simulink model "MMSAR_Sequential2019"  (R2019b)
settings: Solver=VariableStepAuto  StartTime=0.0  StopTime=2.85  RelTol=1e-3
values from neighbouring files (symbols this model uses):
  ADC_input = database_load('EEGdata_ch1.mat',p)'    [MMSeq_main.m]    (also in database_load.m = data(:, epoch))
  C2 = C1*cap_ratio    [MMSeq_main.m]
  Cf_unit_cap = 2    [MMSeq_main.m]
  clk_freq = 2.1*input_BW    (= 537.6)    [MMSeq_main.m]
  clk_period = 1/clk_freq    (= 0.00186011904762)    [MMSeq_main.m]
  comparator_high_offset = 655e-6    (= 0.000655)    [MMSeq_main.m]
  comparator_low_offset = comparator_high_offset    (= 0.000655)    [MMSeq_main.m]
  comparator_noise_on = 1    [MMSeq_main.m]
  comparator_noise_rms = noise_multiplier* 1*sqrt(k*T/C_logic * (2/3))    [MMSeq_main.m]
  comparator_offset_on = 1    [MMSeq_main.m]
  DAC_cap = max([minimum_sampling_cap, minimum_technology_cap, minimum_match_cap_DAC])    [MMSeq_main.m]
  k = 1.38064852e-23    [MMSeq_main.m]
  leak_current = leakage_on *1*10^(-15)    (= 1e-15)    [MMSeq_main.m]
  LNA_bandwidth = 3*input_BW    (= 768)    [MMSeq_main.m]
  LNA_gain = 1000    [MMSeq_main.m]
  LNA_noise_on = 1    [MMSeq_main.m]
  LNA_noise_vector = [pd.random(nb_MAC,1);0]'    [MMSeq_main.m]
  LNA_SR = I_LNA/(nb_activations*MAC_cap)    [MMSeq_main.m]
  MM_attenuation_coeff = 1    [MMSeq_main.m]
  MM_incomplete_transfer_coeff = C1/(C1+C2)    [MMSeq_main.m]
  MM_sampling_noise = noise_multiplier*noise_on*((k*T * C1/(C1+C2)^2) + (k*T*(C1*C2/(C1+C2))/C2^2))    [MMSeq_main.m]
  nb_MAC = 384    [MMSeq_main.m]
  number_of_bits = 6    [MMSeq_main.m]
  sample_time_jitter = 16e-12    (= 1.6e-11)    [MMSeq_main.m]
  sampling_gain = Cs_unit_cap/Cf_unit_cap    [MMSeq_main.m]
  sampling_jitter_on = noise_on    (= 1)    [MMSeq_main.m]
  sim_number = randi(1e6)    [MMSeq_main.m]
  switch_noise_on = noise_on    (= 1)    [MMSeq_main.m]
  switching_noise = noise_multiplier*k*T/(Cf_unit_cap*minimum_sampling_cap)    (= 2.03450520833e-05)    [MMSeq_main.m]
  T = 293    [MMSeq_main.m]
  Vref = 2    [MMSeq_main.m]
  ZOH_delta = 0*Vref/(2^number_of_bits)    (= 0)    [MMSeq_main.m]
libraries: simulink x5, dspsrcs4 x4, simulink_extras x3, dspsigops x2, dspswit3 x2, spsFirstOrderFilterLib x1
settings Model: Creator=mac  LastModifiedBy=mac
settings DataIOCC: SaveFormat=Structure  OutputOption=SpecifiedOutputTimes  OutputTimes=linspace(clk_period*(number_of_bits+5), (nb_channels)*clk_period*nb_MAC+clk_period*(number_of_bits+5),nb_channels+1)
settings DebuggingCC: UnconnectedInputMsg=none  UnconnectedOutputMsg=none

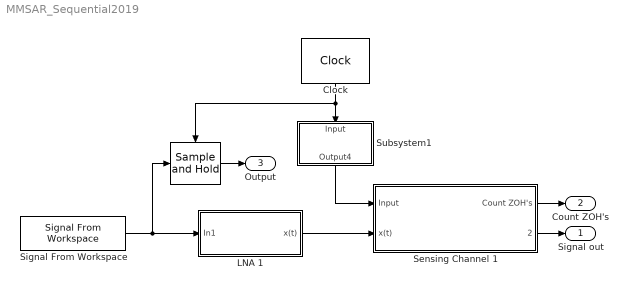
== system MMSAR_Sequential2019 ==
  "           " : dspsigops/Sample and Hold  trig=Rising edge  initCond=0  latchinput=off
  Clock : simulink_extras/Flip Flops/Clock  period=clk_period
  LNA 1 : Subsystem
      mask Display: text(.5, .5, 'LNA', 'horizontalAlignment', 'center', 'verticalAlignment', 'middle')
  Sensing Channel 1 : Subsystem
      mask Display: text(.5, .5, 'Sensing channel', 'horizontalAlignment', 'center', 'verticalAlignment', 'middle')
  Signal From Workspace : dspsrcs4/Signal From Workspace  X=ADC_input  Ts=clk_period  nsamps=1  OutputAfterFinalValue=Cyclic repetition  ignoreOrWarnInputAndFrameLengths=off  OutputFrames=off
  Subsystem1 : Subsystem
      mask Display: text(.5, .5, 'Clocking block', 'horizontalAlignment', 'center', 'verticalAlignment', 'middle')
  Signal out : Outport
  Count ZOH's : Outport  Port=2
  Output : Outport  Port=3
  wires:
  Sensing Channel 1/1(Count ZOH's) -> Count ZOH's/1
  Subsystem1/1(Output4) -> Sensing Channel 1/1(Input)
  Signal From Workspace/1 -> "           "/1, LNA 1/1(In1)
  LNA 1/1(x(t)) -> Sensing Channel 1/2(x(t))
  Clock/1 -> Subsystem1/1(Input), "           "/Trigger
  Sensing Channel 1/2(" ") -> Signal out/1
  "           "/1 -> Output/1

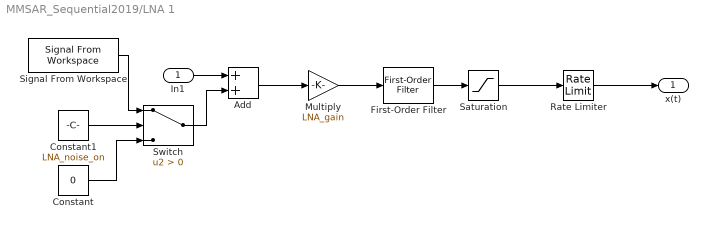
== system MMSAR_Sequential2019/LNA 1 ==
  In1 : Inport
  Add : Sum
  Constant : Constant  Value=0
  Constant1 : Constant  Value=LNA_noise_on
  First-Order Filter : spsFirstOrderFilterLib/First-Order Filter  FilterType=Lowpass  Tc=1/(LNA_bandwidth*2*pi)  Ts=0  Initialize=on  Vac_Init=[0, 0, 60]  Vdc_Init=(LNA_noise_vector(1,1)+double(ADC_input(1,1)))*LNA_gain  PlotResponse=off  FreqRange="[0,  200,  1]"
  Multiply : Gain  Gain=LNA_gain
  Rate Limiter : RateLimiter  RisingSlewLimit=LNA_SR  FallingSlewLimit=-LNA_SR  SampleTimeMode=inherited  InitialCondition=(LNA_noise_vector(1,1)+double(ADC_input(1,1)))*LNA_gain
  Saturation : Saturate  UpperLimit=Vref  LowerLimit=0
  Signal From Workspace : dspsrcs4/Signal From Workspace  X=LNA_noise_vector  Ts=clk_period  nsamps=1  OutputAfterFinalValue=Cyclic repetition  ignoreOrWarnInputAndFrameLengths=off  OutputFrames=off
  Switch : Switch  Criteria=u2 > Threshold
  x(t) : Outport
  wires:
  In1/1 -> Add/1
  Add/1 -> Multiply/1
  Constant/1 -> Switch/3
  Constant1/1 -> Switch/2
  Switch/1 -> Add/2
  Multiply/1 -> First-Order Filter/1
  Signal From Workspace/1 -> Switch/1
  First-Order Filter/1 -> Saturation/1
  Saturation/1 -> Rate Limiter/1
  Rate Limiter/1 -> x(t)/1

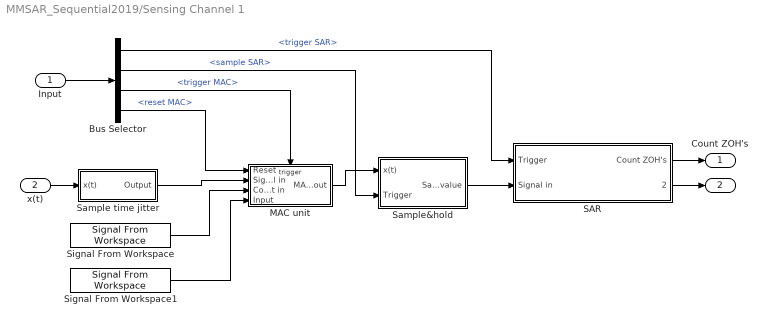
== system MMSAR_Sequential2019/Sensing Channel 1 ==
  Input : Inport
  x(t) : Inport  Port=2
  Bus Selector : BusSelector  OutputSignals=trigger SAR,sample SAR,trigger MAC,reset MAC
  MAC unit : Subsystem
      mask Display: text(.5, .5, 'MAC unit', 'horizontalAlignment', 'center', 'verticalAlignment', 'middle')
  SAR : Subsystem
      mask Display: text(.5, .5, 'ZOH SAR', 'horizontalAlignment', 'center', 'verticalAlignment', 'middle')
  Sample time jitter : Subsystem
      mask Display: text(.5, .5, 'Sampling jitter', 'horizontalAlignment', 'center', 'verticalAlignment', 'middle')
  Sample&hold : Subsystem
      mask Display: text(.5, .5, 'Sample & hold', 'horizontalAlignment', 'center', 'verticalAlignment', 'middle')
  Signal From Workspace : dspsrcs4/Signal From Workspace  X=sensing_matrix  Ts=clk_period  nsamps=1  OutputAfterFinalValue=Setting to zero  ignoreOrWarnInputAndFrameLengths=off  OutputFrames=off
  Signal From Workspace1 : dspsrcs4/Signal From Workspace  X=sensingOrderMatrix  Ts=clk_period  nsamps=1  OutputAfterFinalValue=Cyclic repetition  ignoreOrWarnInputAndFrameLengths=off  OutputFrames=off
  Count ZOH's : Outport
  " " : Outport  Port=2
  wires:
  SAR/2(" ") -> " "/1
  MAC unit/1(MAC_out) -> Sample&hold/1(x(t))
  Sample&hold/1(Sampled value) -> SAR/2(Signal in)
  Input/1 -> Bus Selector/1
  Bus Selector/4 -> MAC unit/1(Reset)  "<reset MAC>"
  Bus Selector/2 -> Sample&hold/2(Trigger)  "<sample SAR>"
  Bus Selector/1 -> SAR/1(Trigger)  "<trigger SAR>"
  Signal From Workspace/1 -> MAC unit/3(Coefficient in)
  Bus Selector/3 -> MAC unit/Trigger  "<trigger MAC>"
  SAR/1(Count ZOH's) -> Count ZOH's/1
  x(t)/1 -> Sample time jitter/1(x(t))
  Sample time jitter/1(Output) -> MAC unit/2(Signal in)
  Signal From Workspace1/1 -> MAC unit/4(Input)

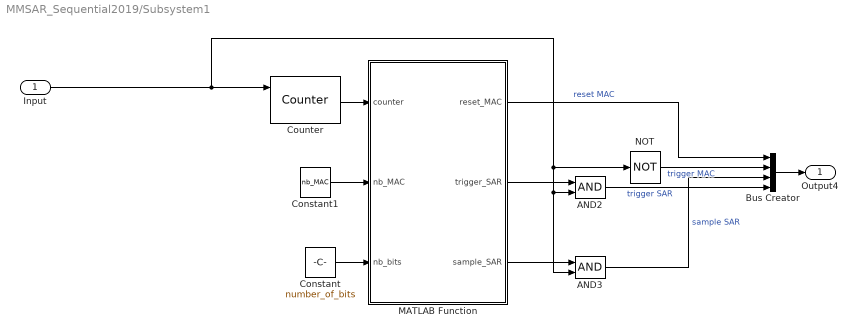
== system MMSAR_Sequential2019/Subsystem1 ==
  Input : Inport
  AND2 : Logic  IconShape=distinctive  AllPortsSameDT=off  OutDataTypeStr=boolean
  AND3 : Logic  IconShape=distinctive  AllPortsSameDT=off  OutDataTypeStr=boolean
  Bus Creator : BusCreator  Inputs=4
  Constant : Constant  Value=number_of_bits
  Constant1 : Constant  Value=nb_MAC
  Counter : dspswit3/Counter  Direction=Up  CountEvent=Rising edge  CounterSize=User defined  MaxCount=nb_MAC-1  InitialCount=0  Output=Count  HitValue=32  ResetInput=on  SamplesPerFrame=1  Ts=1  CntDtype=double  HitDtype=Logical
  MATLAB Function : MATLAB Function  TreatAsAtomicUnit=on
  NOT : Logic  Operator=NOT  IconShape=distinctive  AllPortsSameDT=off  OutDataTypeStr=boolean
  Output4 : Outport
  wires:
  Counter/1 -> MATLAB Function/1(counter)
  Constant1/1 -> MATLAB Function/2(nb_MAC)
  Input/1 -> Counter/1, NOT/1, AND3/2, AND2/2
  AND2/1 -> Bus Creator/4  "trigger SAR"
  AND3/1 -> Bus Creator/3  "sample SAR"
  MATLAB Function/3(sample_SAR) -> AND3/1
  MATLAB Function/2(trigger_SAR) -> AND2/1
  MATLAB Function/1(reset_MAC) -> Bus Creator/1  "reset MAC"
  Bus Creator/1 -> Output4/1
  Constant/1 -> MATLAB Function/3(nb_bits)
  NOT/1 -> Bus Creator/2  "trigger MAC"

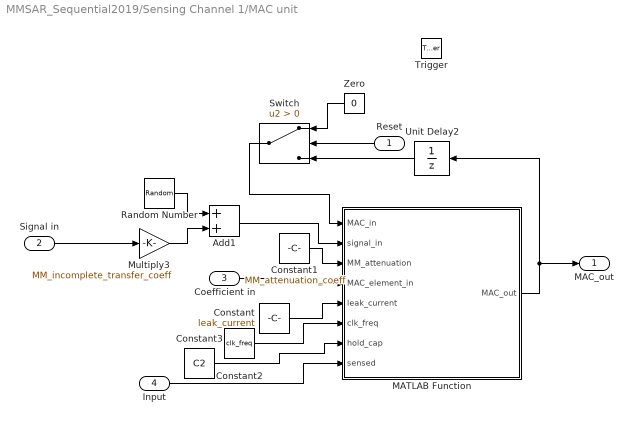
== system MMSAR_Sequential2019/Sensing Channel 1/MAC unit ==
  Reset : Inport
  Signal in : Inport  Port=2
  Coefficient in : Inport  Port=3
  Input : Inport  Port=4
  Trigger : TriggerPort  VariantControl=Variant  PortDimensions=1
  Add1 : Sum
  Constant : Constant  Value=leak_current
  Constant1 : Constant  Value=MM_attenuation_coeff
  Constant2 : Constant  Value=clk_freq
  Constant3 : Constant  Value=C2
  MATLAB Function : MATLAB Function  TreatAsAtomicUnit=on
  Multiply3 : Gain  Gain=MM_incomplete_transfer_coeff
  Random Number : RandomNumber  Variance=MM_sampling_noise  Seed=1*sim_number
  Switch : Switch  Criteria=u2 > Threshold
  Unit Delay2 : UnitDelay  InitialCondition=1  SampleTime=-1  HasFrameUpgradeWarning=on
  Zero : Constant  Value=0  OutDataTypeStr=Inherit: Inherit via back propagation
  MAC_out : Outport
  wires:
  Multiply3/1 -> Add1/2
  Random Number/1 -> Add1/1
  Constant1/1 -> MATLAB Function/3(MM_attenuation)
  MATLAB Function/1(MAC_out) -> Unit Delay2/1, MAC_out/1
  Add1/1 -> MATLAB Function/2(signal_in)
  Coefficient in/1 -> MATLAB Function/4(MAC_element_in)
  Switch/1 -> MATLAB Function/1(MAC_in)
  Reset/1 -> Switch/2
  Unit Delay2/1 -> Switch/3
  Zero/1 -> Switch/1
  Signal in/1 -> Multiply3/1
  Constant/1 -> MATLAB Function/5(leak_current)
  Constant3/1 -> MATLAB Function/7(hold_cap)
  Constant2/1 -> MATLAB Function/6(clk_freq)
  Input/1 -> MATLAB Function/8(sensed)

== system MMSAR_Sequential2019/Sensing Channel 1/SAR ==
  Trigger : Inport
  Signal in : Inport  Port=2
  "           " : dspsigops/Sample and Hold  trig=Rising edge  initCond=0  latchinput=off
  Constant : Constant  Value=Vref
  Constant1 : Constant  Value=number_of_bits
  DAC : Subsystem  TreatAsAtomicUnit=on
      mask Display: text(.5, .5, 'DAC', 'horizontalAlignment', 'center', 'verticalAlignment', 'middle')
  SAR : Subsystem  TreatAsAtomicUnit=on
      mask Display: text(.5, .5, 'SAR', 'horizontalAlignment', 'center', 'verticalAlignment', 'middle')
  ZOH+comparator : Subsystem
      mask Display: text(.5, .5, 'Comparator', 'horizontalAlignment', 'center', 'verticalAlignment', 'middle')
  Count ZOH's : Outport
  " " : Outport  Port=2
  wires:
  SAR/2(SAR_done) -> "           "/Trigger
  ZOH+comparator/3(Output) -> Count ZOH's/1
  SAR/3(Output_code) -> DAC/3(Input_code)
  "           "/1 -> " "/1  "SAR output"
  Constant/1 -> DAC/2(Vref)
  ZOH+comparator/1(Output2) -> SAR/1(Comparator_in)
  Signal in/1 -> ZOH+comparator/1(Signal in)  "SAR in"
  Constant1/1 -> SAR/3(Number of bits), DAC/1(NOB)
  DAC/1(y) -> ZOH+comparator/2(DAC in), "           "/1
  ZOH+comparator/2(Output1) -> SAR/2(ZOH)
  SAR/1(Output) -> ZOH+comparator/3(Input)
  Trigger/1 -> SAR/Trigger, ZOH+comparator/4(Clk)

== system MMSAR_Sequential2019/Sensing Channel 1/Sample time jitter ==
  x(t) : Inport
  Add : Sum
  Constant : Constant  Value=sampling_jitter_on
  Derivative : Derivative
  Multiply : Gain  Gain=sample_time_jitter
  Product : Product
  Random Number : RandomNumber  Seed=2*sim_number  SampleTime=clk_period
  Switch : Switch  Criteria=u2 > Threshold
  Zero-Order Hold : ZeroOrderHold  SampleTime=-1
  Output : Outport
  wires:
  Random Number/1 -> Zero-Order Hold/1
  x(t)/1 -> Add/1, Switch/3, Derivative/1
  Zero-Order Hold/1 -> Multiply/1
  Product/1 -> Add/2
  Derivative/1 -> Product/1
  Multiply/1 -> Product/2
  Switch/1 -> Output/1
  Add/1 -> Switch/1
  Constant/1 -> Switch/2

== system MMSAR_Sequential2019/Sensing Channel 1/Sample&hold ==
  x(t) : Inport
  Trigger : Inport  Port=2
  Sample switch noise : Subsystem  TreatAsAtomicUnit=on
  Sampled value : Outport
  wires:
  Trigger/1 -> Sample switch noise/Trigger
  Sample switch noise/1(y(t)) -> Sampled value/1  "Sampled value"
  x(t)/1 -> Sample switch noise/1(Input)

== system MMSAR_Sequential2019/Sensing Channel 1/SAR/DAC ==
  NOB : Inport
  Vref : Inport  Port=2
  Input_code : Inport  Port=3
  DAC : MATLAB Function  TreatAsAtomicUnit=on
  y : Outport
  wires:
  NOB/1 -> DAC/2(number_of_bits)
  Vref/1 -> DAC/3(Vref)
  DAC/1(out) -> y/1
  Input_code/1 -> DAC/1(input_code)

== system MMSAR_Sequential2019/Sensing Channel 1/SAR/SAR ==
  Comparator_in : Inport  LatchByDelayingOutsideSignal=on
  ZOH : Inport  Port=2  LatchByDelayingOutsideSignal=on
  Number of bits : Inport  Port=3
  Trigger : TriggerPort  VariantControl=Variant
  SAR : MATLAB Function  TreatAsAtomicUnit=on
  Unit Delay : UnitDelay  SampleTime=-1  HasFrameUpgradeWarning=on
  Unit Delay1 : UnitDelay  SampleTime=-1  HasFrameUpgradeWarning=on
  Output : Outport
  SAR_done : Outport  Port=2  InitialOutput=0
  Output_code : Outport  Port=3  InitialOutput=zeros(number_of_bits, 1)
      settings: VarSizeSig=Yes
  wires:
  Number of bits/1 -> SAR/4(number_of_bits)
  Comparator_in/1 -> SAR/3(comparator_in)
  Unit Delay1/1 -> SAR/2(cycle_in)
  SAR/3(output_code) -> Output_code/1
  Unit Delay/1 -> SAR/1(input_code_decimal)
  SAR/1(output_code_decimal) -> Unit Delay/1
  SAR/4(done) -> SAR_done/1
  ZOH/1 -> SAR/5(ZOH_true)
  SAR/2(cycle_out) -> Output/1, Unit Delay1/1

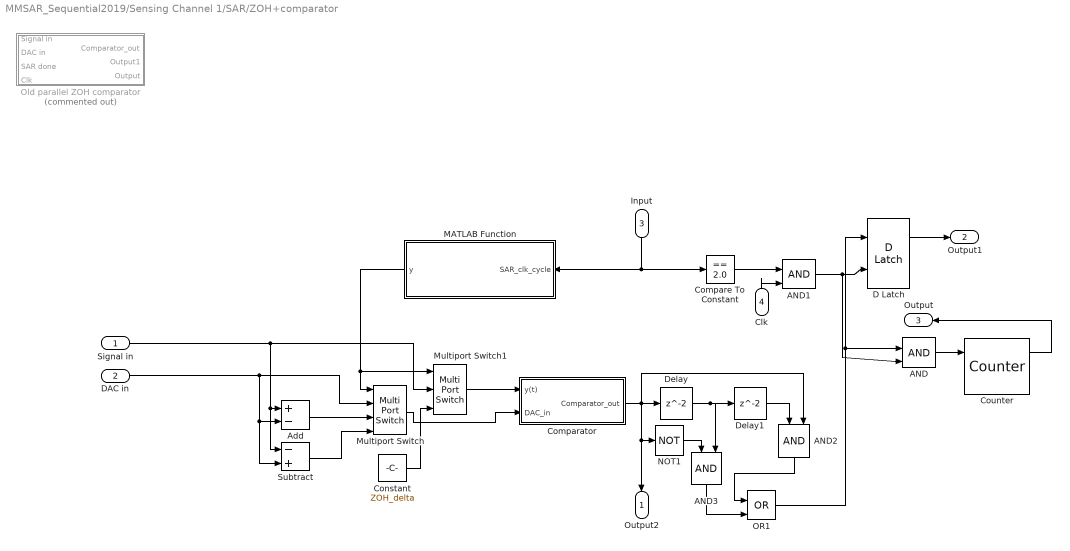
== system MMSAR_Sequential2019/Sensing Channel 1/SAR/ZOH+comparator ==
  Signal in : Inport
  DAC in : Inport  Port=2
  Input : Inport  Port=3
  Clk : Inport  Port=4
  AND{,1..3} (4 alike) : Logic  IconShape=distinctive  AllPortsSameDT=off  OutDataTypeStr=boolean
  Add : Sum  Inputs=+-
  Comparator : Subsystem  TreatAsAtomicUnit=on
      mask Display: text(.5, .5, 'Comparator', 'horizontalAlignment', 'center', 'verticalAlignment', 'middle')
  Compare To Constant : simulink/Logic and Bit Operations/Compare To Constant  relop===  const=2.0  OutDataTypeStr=boolean
  Constant : Constant  Value=ZOH_delta
  Counter : dspswit3/Counter  Direction=Up  CountEvent=Rising edge  CounterSize=User defined  MaxCount=255  InitialCount=0  Output=Count and Hit  HitValue=32  ResetInput=on  SamplesPerFrame=1  Ts=1  CntDtype=double  HitDtype=Logical
  D Latch : simulink_extras/Flip Flops/D Latch
      settings: SourceProductBaseCode=SL
  Delay : Delay
  Delay1 : Delay
  MATLAB Function : MATLAB Function  TreatAsAtomicUnit=on
  Multiport Switch : MultiPortSwitch
  Multiport Switch1 : MultiPortSwitch  Inputs=2  DiagnosticForDefault=None
  NOT1 : Logic  Operator=NOT  IconShape=distinctive  AllPortsSameDT=off  OutDataTypeStr=boolean
  OR1 : Logic  Operator=OR  IconShape=distinctive  AllPortsSameDT=off  OutDataTypeStr=boolean
  Old parallel ZOH comparator : Subsystem  Commented=on
      mask Display: text(.5, .5, 'ZOH comparator', 'horizontalAlignment', 'center', 'verticalAlignment', 'middle')
  Subtract : Sum  Inputs=-+
  Output2 : Outport
  Output1 : Outport  Port=2
  Output : Outport  Port=3
  wires:
  Delay/1 -> Delay1/1, AND3/2
  Constant/1 -> Multiport Switch1/3
  DAC in/1 -> Multiport Switch/2, Subtract/2, Add/2
  D Latch/1 -> Output1/1
  Add/1 -> Multiport Switch/3
  Signal in/1 -> Subtract/1, Add/1, Multiport Switch1/2
  Multiport Switch1/1 -> Comparator/1(y(t))
  Comparator/1(Comparator_out) -> Delay/1, AND2/2, Output2/1, NOT1/1
  Delay1/1 -> AND2/1
  MATLAB Function/1(y) -> Multiport Switch1/1, Multiport Switch/1
  Input/1 -> Compare To Constant/1, MATLAB Function/1(SAR_clk_cycle)
  Compare To Constant/1 -> AND1/1
  Counter/1 -> Output/1
  Multiport Switch/1 -> Comparator/2(DAC_in)
  Subtract/1 -> Multiport Switch/4
  NOT1/1 -> AND3/1
  AND3/1 -> OR1/2
  AND2/1 -> OR1/1
  Clk/1 -> AND1/2
  OR1/1 -> AND/1, D Latch/1
  AND1/1 -> AND/2, D Latch/2
  AND/1 -> Counter/1

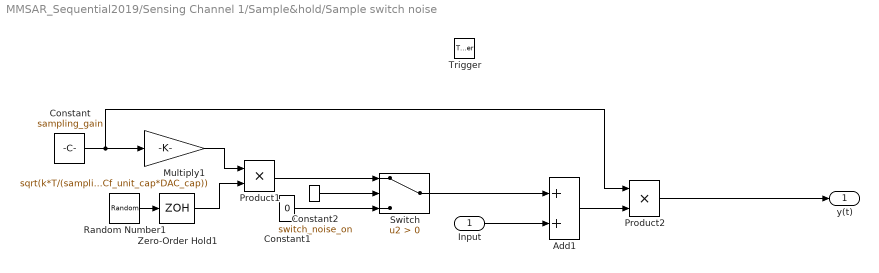
== system MMSAR_Sequential2019/Sensing Channel 1/Sample&hold/Sample switch noise ==
  Input : Inport
  Trigger : TriggerPort  VariantControl=Variant
  Add1 : Sum
  Constant : Constant  Value=sampling_gain
  Constant1 : Constant  Value=0
  Constant2 : Constant  Value=switch_noise_on
  Multiply1 : Gain  Gain=sqrt(k*T/(sampling_gain*Cf_unit_cap*DAC_cap))  OutDataTypeStr=Inherit: Same as input
  Product1 : Product
  Product2 : Product
  Random Number1 : RandomNumber  Variance=switching_noise  Seed=3*sim_number
  Switch : Switch  Criteria=u2 > Threshold
  Zero-Order Hold1 : ZeroOrderHold  SampleTime=-1
  y(t) : Outport
  wires:
  Product2/1 -> y(t)/1
  Random Number1/1 -> Zero-Order Hold1/1
  Multiply1/1 -> Product1/1
  Add1/1 -> Product2/2
  Constant/1 -> Product2/1, Multiply1/1
  Constant2/1 -> Switch/2
  Constant1/1 -> Switch/3
  Product1/1 -> Switch/1
  Zero-Order Hold1/1 -> Product1/2
  Switch/1 -> Add1/1
  Input/1 -> Add1/2

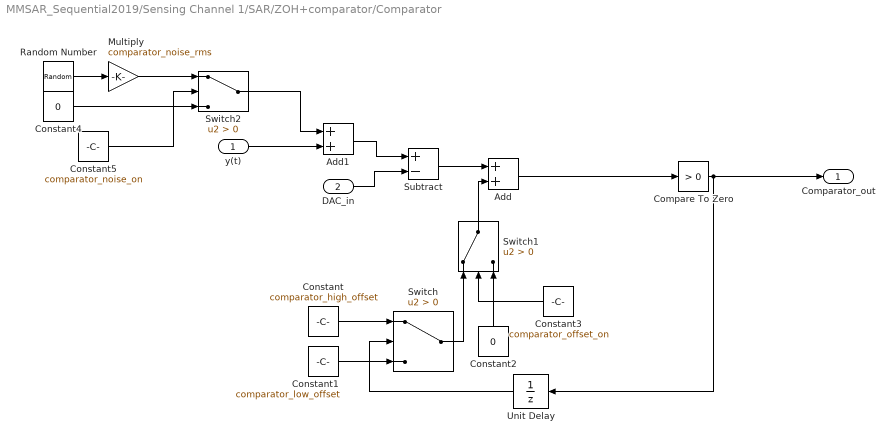
== system MMSAR_Sequential2019/Sensing Channel 1/SAR/ZOH+comparator/Comparator ==
  y(t) : Inport
  DAC_in : Inport  Port=2
  Add : Sum
  Add1 : Sum
  Compare To Zero : simulink/Logic and Bit Operations/Compare To Zero  relop=>  OutDataTypeStr=boolean
  Constant : Constant  Value=comparator_high_offset
  Constant1 : Constant  Value=comparator_low_offset
  Constant2 : Constant  Value=0
  Constant3 : Constant  Value=comparator_offset_on
  Constant4 : Constant  Value=0
  Constant5 : Constant  Value=comparator_noise_on
  Multiply : Gain  Gain=comparator_noise_rms
  Random Number : RandomNumber  Seed=4*sim_number  SampleTime=1/clk_freq
  Subtract : Sum  Inputs=+-
  Switch : Switch  Criteria=u2 > Threshold
  Switch1 : Switch  Criteria=u2 > Threshold
  Switch2 : Switch  Criteria=u2 > Threshold
  Unit Delay : UnitDelay  SampleTime=-1  HasFrameUpgradeWarning=on
  Comparator_out : Outport
  wires:
  Switch/1 -> Switch1/1
  Subtract/1 -> Add/1
  Constant/1 -> Switch/1
  Constant2/1 -> Switch1/3
  Add/1 -> Compare To Zero/1
  Switch1/1 -> Add/2
  Constant3/1 -> Switch1/2
  Unit Delay/1 -> Switch/2
  Constant1/1 -> Switch/3
  DAC_in/1 -> Subtract/2
  Add1/1 -> Subtract/1
  y(t)/1 -> Add1/2
  Random Number/1 -> Multiply/1
  Switch2/1 -> Add1/1
  Multiply/1 -> Switch2/1
  Constant4/1 -> Switch2/3
  Constant5/1 -> Switch2/2
  Compare To Zero/1 -> Unit Delay/1, Comparator_out/1

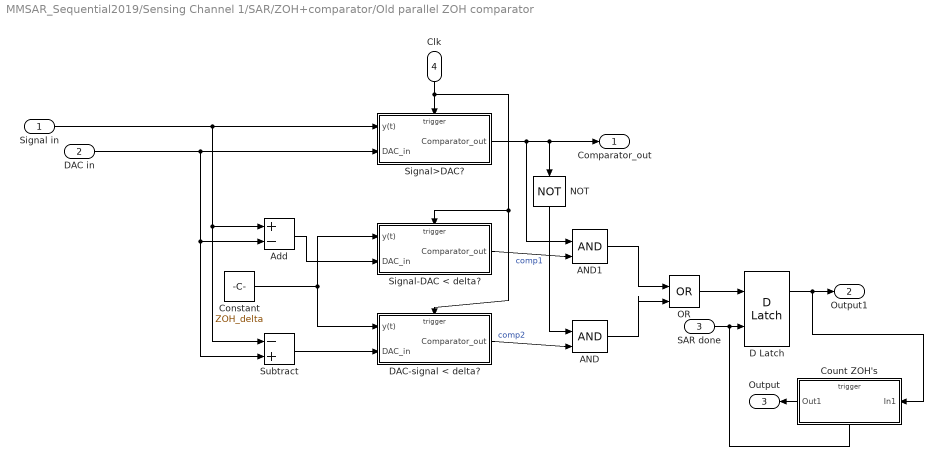
== system MMSAR_Sequential2019/Sensing Channel 1/SAR/ZOH+comparator/Old parallel ZOH comparator ==
  Signal in : Inport
  DAC in : Inport  Port=2
  SAR done : Inport  Port=3
  Clk : Inport  Port=4
  " DAC-signal < delta?" : Subsystem  TreatAsAtomicUnit=on
      mask Display: text(.5, .5, 'Comparator', 'horizontalAlignment', 'center', 'verticalAlignment', 'middle')
  AND : Logic  IconShape=distinctive  AllPortsSameDT=off  OutDataTypeStr=boolean
  AND1 : Logic  IconShape=distinctive  AllPortsSameDT=off  OutDataTypeStr=boolean
  Add : Sum  Inputs=+-
  Constant : Constant  Value=ZOH_delta
  Count ZOH's : Subsystem
  D Latch : simulink_extras/Flip Flops/D Latch
      settings: SourceProductBaseCode=SL
  NOT : Logic  Operator=NOT  IconShape=distinctive  AllPortsSameDT=off  OutDataTypeStr=boolean
  OR : Logic  Operator=OR  IconShape=distinctive  AllPortsSameDT=off  OutDataTypeStr=boolean
  Signal-DAC < delta? : Subsystem  TreatAsAtomicUnit=on
      mask Display: text(.5, .5, 'Comparator', 'horizontalAlignment', 'center', 'verticalAlignment', 'middle')
  Signal>DAC? : Subsystem  TreatAsAtomicUnit=on
      mask Display: text(.5, .5, 'Comparator', 'horizontalAlignment', 'center', 'verticalAlignment', 'middle')
  Subtract : Sum  Inputs=-+
  Comparator_out : Outport
  Output1 : Outport  Port=2
  Output : Outport  Port=3
  wires:
  Signal>DAC?/1(Comparator_out) -> NOT/1, Comparator_out/1, AND1/1
  AND1/1 -> OR/1
  Subtract/1 -> " DAC-signal < delta?"/2(DAC_in)
  Signal in/1 -> Add/1, Subtract/1, Signal>DAC?/1(y(t))
  Clk/1 -> Signal>DAC?/Trigger, Signal-DAC < delta?/Trigger, " DAC-signal < delta?"/Trigger
  AND/1 -> OR/2
  " DAC-signal < delta?"/1(Comparator_out) -> AND/2  "comp2"
  Signal-DAC < delta?/1(Comparator_out) -> AND1/2  "comp1"
  Add/1 -> Signal-DAC < delta?/2(DAC_in)
  DAC in/1 -> Subtract/2, Add/2, Signal>DAC?/2(DAC_in)
  Constant/1 -> Signal-DAC < delta?/1(y(t)), " DAC-signal < delta?"/1(y(t))
  NOT/1 -> AND/1
  OR/1 -> D Latch/1
  D Latch/1 -> Count ZOH's/1(In1), Output1/1
  Count ZOH's/1(Out1) -> Output/1
  SAR done/1 -> Count ZOH's/Trigger, D Latch/2

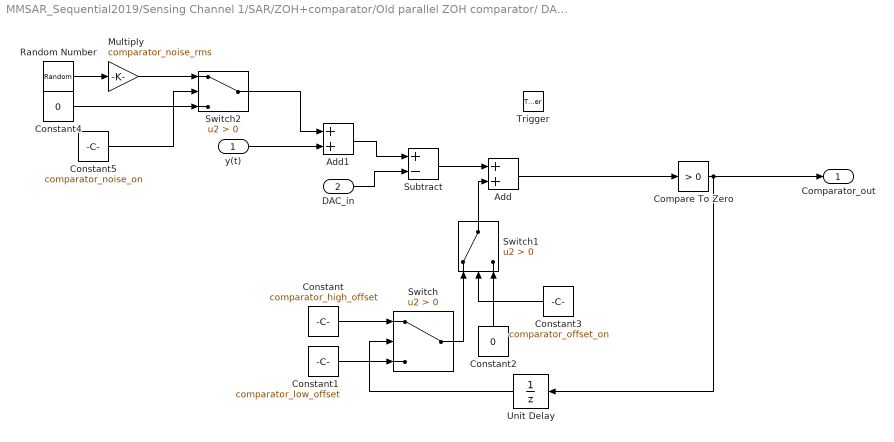
== system MMSAR_Sequential2019/Sensing Channel 1/SAR/ZOH+comparator/Old parallel ZOH comparator/ DAC-signal < delta? ==
  y(t) : Inport
  DAC_in : Inport  Port=2
  Trigger : TriggerPort  VariantControl=Variant
  Add : Sum
  Add1 : Sum
  Compare To Zero : simulink/Logic and Bit Operations/Compare To Zero  relop=>  OutDataTypeStr=boolean
  Constant : Constant  Value=comparator_high_offset
  Constant1 : Constant  Value=comparator_low_offset
  Constant2 : Constant  Value=0
  Constant3 : Constant  Value=comparator_offset_on
  Constant4 : Constant  Value=0
  Constant5 : Constant  Value=comparator_noise_on
  Multiply : Gain  Gain=comparator_noise_rms
  Random Number : RandomNumber
  Subtract : Sum  Inputs=+-
  Switch : Switch  Criteria=u2 > Threshold
  Switch1 : Switch  Criteria=u2 > Threshold
  Switch2 : Switch  Criteria=u2 > Threshold
  Unit Delay : UnitDelay  SampleTime=-1  HasFrameUpgradeWarning=on
  Comparator_out : Outport
  wires:
  Switch/1 -> Switch1/1
  Subtract/1 -> Add/1
  Constant/1 -> Switch/1
  Constant2/1 -> Switch1/3
  Add/1 -> Compare To Zero/1
  Switch1/1 -> Add/2
  Compare To Zero/1 -> Unit Delay/1, Comparator_out/1
  Constant3/1 -> Switch1/2
  Unit Delay/1 -> Switch/2
  Constant1/1 -> Switch/3
  DAC_in/1 -> Subtract/2
  Add1/1 -> Subtract/1
  y(t)/1 -> Add1/2
  Random Number/1 -> Multiply/1
  Switch2/1 -> Add1/1
  Multiply/1 -> Switch2/1
  Constant4/1 -> Switch2/3
  Constant5/1 -> Switch2/2

== system MMSAR_Sequential2019/Sensing Channel 1/SAR/ZOH+comparator/Old parallel ZOH comparator/Count ZOH's ==
  In1 : Inport
  Trigger : TriggerPort  VariantControl=Variant  PortDimensions=1
  Add : Sum  AccumDataTypeStr=double  OutDataTypeStr=double
  Unit Delay : UnitDelay  SampleTime=-1  HasFrameUpgradeWarning=on
  Out1 : Outport
  wires:
  In1/1 -> Add/1
  Add/1 -> Unit Delay/1, Out1/1
  Unit Delay/1 -> Add/2

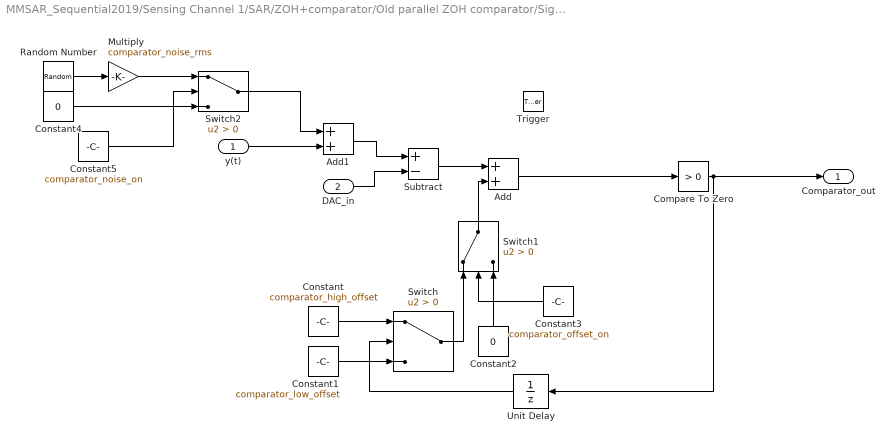
== system MMSAR_Sequential2019/Sensing Channel 1/SAR/ZOH+comparator/Old parallel ZOH comparator/Signal-DAC < delta? ==
  y(t) : Inport
  DAC_in : Inport  Port=2
  Trigger : TriggerPort  VariantControl=Variant
  Add : Sum
  Add1 : Sum
  Compare To Zero : simulink/Logic and Bit Operations/Compare To Zero  relop=>  OutDataTypeStr=boolean
  Constant : Constant  Value=comparator_high_offset
  Constant1 : Constant  Value=comparator_low_offset
  Constant2 : Constant  Value=0
  Constant3 : Constant  Value=comparator_offset_on
  Constant4 : Constant  Value=0
  Constant5 : Constant  Value=comparator_noise_on
  Multiply : Gain  Gain=comparator_noise_rms
  Random Number : RandomNumber
  Subtract : Sum  Inputs=+-
  Switch : Switch  Criteria=u2 > Threshold
  Switch1 : Switch  Criteria=u2 > Threshold
  Switch2 : Switch  Criteria=u2 > Threshold
  Unit Delay : UnitDelay  SampleTime=-1  HasFrameUpgradeWarning=on
  Comparator_out : Outport
  wires:
  Switch/1 -> Switch1/1
  Subtract/1 -> Add/1
  Constant/1 -> Switch/1
  Constant2/1 -> Switch1/3
  Add/1 -> Compare To Zero/1
  Switch1/1 -> Add/2
  Compare To Zero/1 -> Unit Delay/1, Comparator_out/1
  Constant3/1 -> Switch1/2
  Unit Delay/1 -> Switch/2
  Constant1/1 -> Switch/3
  DAC_in/1 -> Subtract/2
  Add1/1 -> Subtract/1
  y(t)/1 -> Add1/2
  Random Number/1 -> Multiply/1
  Switch2/1 -> Add1/1
  Multiply/1 -> Switch2/1
  Constant4/1 -> Switch2/3
  Constant5/1 -> Switch2/2

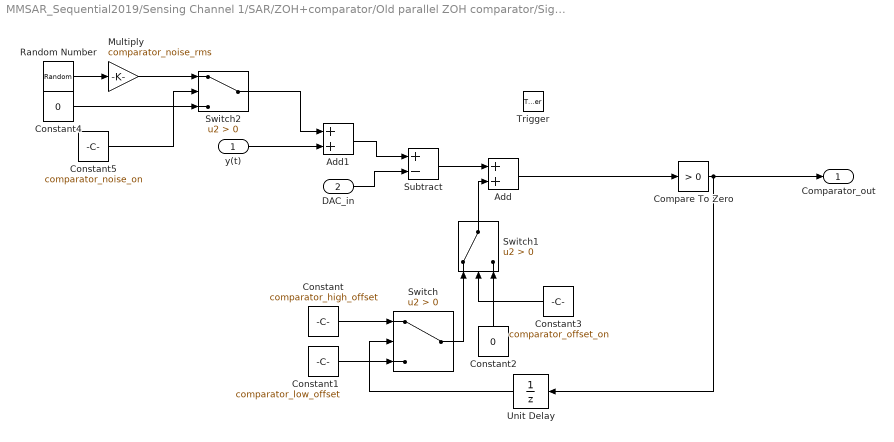
== system MMSAR_Sequential2019/Sensing Channel 1/SAR/ZOH+comparator/Old parallel ZOH comparator/Signal>DAC? ==
  y(t) : Inport
  DAC_in : Inport  Port=2
  Trigger : TriggerPort  VariantControl=Variant
  Add : Sum
  Add1 : Sum
  Compare To Zero : simulink/Logic and Bit Operations/Compare To Zero  relop=>  OutDataTypeStr=boolean
  Constant : Constant  Value=comparator_high_offset
  Constant1 : Constant  Value=comparator_low_offset
  Constant2 : Constant  Value=0
  Constant3 : Constant  Value=comparator_offset_on
  Constant4 : Constant  Value=0
  Constant5 : Constant  Value=comparator_noise_on
  Multiply : Gain  Gain=comparator_noise_rms
  Random Number : RandomNumber
  Subtract : Sum  Inputs=+-
  Switch : Switch  Criteria=u2 > Threshold
  Switch1 : Switch  Criteria=u2 > Threshold
  Switch2 : Switch  Criteria=u2 > Threshold
  Unit Delay : UnitDelay  SampleTime=-1  HasFrameUpgradeWarning=on
  Comparator_out : Outport
  wires:
  Switch/1 -> Switch1/1
  Subtract/1 -> Add/1
  Constant/1 -> Switch/1
  Constant2/1 -> Switch1/3
  Add/1 -> Compare To Zero/1
  Switch1/1 -> Add/2
  Compare To Zero/1 -> Unit Delay/1, Comparator_out/1
  Constant3/1 -> Switch1/2
  Unit Delay/1 -> Switch/2
  Constant1/1 -> Switch/3
  DAC_in/1 -> Subtract/2
  Add1/1 -> Subtract/1
  y(t)/1 -> Add1/2
  Random Number/1 -> Multiply/1
  Switch2/1 -> Add1/1
  Multiply/1 -> Switch2/1
  Constant4/1 -> Switch2/3
  Constant5/1 -> Switch2/2

== matlab function MMSAR_Sequential2019/Sensing Channel 1/SAR/ZOH+comparator/MATLAB Function ==
  data: SAR_clk_cycle input; y output
function y = fcn(SAR_clk_cycle)
    if (SAR_clk_cycle)==0
        y = 2;
    elseif (SAR_clk_cycle)==1
        y=3;
    else
        y=1;
    end
end

== matlab function MMSAR_Sequential2019/Sensing Channel 1/SAR/DAC/DAC ==
  data: input_code input size=number_of_bits; out output double size=1; number_of_bits input; Vref input
function out = fcn(input_code, number_of_bits, Vref)
out = Vref/(2^number_of_bits) * (bi2de(input_code.', 'left-msb'));
end

== matlab function MMSAR_Sequential2019/Sensing Channel 1/SAR/SAR/SAR ==
  data: output_code_decimal output size=1; cycle_out output size=1; output_code output size=number_of_bits; input_code_decimal input; cycle_in input; comparator_in input; number_of_bits input; done output; ZOH_true input
function [output_code_decimal, cycle_out, output_code, done] = fcn(input_code_decimal, cycle_in, comparator_in, number_of_bits, ZOH_true)

    input_code = de2bi(input_code_decimal, 'left-msb');
    output_code = [zeros(number_of_bits-size(input_code.',1),1); input_code.'];
    cycle_out = cycle_in + 1;
    done = 0;

    if (cycle_in < 2)
        
        % Wait for ZOH to be determined
        
    elseif (cycle_in == 2)
        % Reset output code, start SA algorithm unless ZOH
        if (~ZOH_true)
            output_code = zeros(number_of_bits,1);
            output_code(1, 1) = 1;
        end
        
    elseif (cycle_in == number_of_bits+2)
        % Finish SA algorithm unless ZOH, set done & reset output_cycle
        done = 1;
        if (~ZOH_true)
            output_code(number_of_bits,1) = comparator_in;
        end
        cycle_out = 0;
    else
        % Continue SA algorithm unless ZOH
        if (~ZOH_true)
            if (comparator_in == 0)
                output_code(cycle_in-2,1) = 0;
            end

            output_code(cycle_in-1,1) = 1;
        end
        
    end
    
    output_code_decimal_temp = bi2de(output_code.', 'left-msb');
    output_code_decimal = output_code_decimal_temp(1,1);
end

== matlab function MMSAR_Sequential2019/Subsystem1/MATLAB Function ==
  data: counter input; nb_MAC input; reset_MAC output; trigger_SAR output; sample_SAR output; nb_bits input
function [reset_MAC, trigger_SAR, sample_SAR] = control_logic(counter, nb_MAC, nb_bits)

    reset_MAC = 0;
    trigger_SAR = 0;
    sample_SAR = 0;
    
    if (counter==0)
        reset_MAC = 1;
        sample_SAR = 1;
    end
    if (counter<nb_bits+3)
        trigger_SAR = 1;
    end
    if (counter == nb_MAC-1)
        sample_SAR = 1;
    end

   
end

== matlab function MMSAR_Sequential2019/Sensing Channel 1/MAC unit/MATLAB Function ==
  data: MAC_in input; signal_in input; MAC_out output; MM_attenuation input; MAC_element_in input; leak_current input; clk_freq input; hold_cap input; sensed input
function MAC_out = fcn(MAC_in, signal_in, MM_attenuation, MAC_element_in, leak_current, clk_freq, hold_cap, sensed)

if (MAC_element_in == 0)
    MAC_out = MAC_in;
else 
    MAC_out = signal_in*MAC_element_in + MM_attenuation*MAC_in;
end
if sensed==0 % Only leak if not sensed yet (in real implementation, it would be digitized. In this model, digitization always happens after full amount of cycles)
    MAC_out = max(0,MAC_out - leak_current/(clk_freq*hold_cap));
end
% MAC_out = MAC_out - leak_current/(clk_freq*hold_cap);
end
